simulink model "model"  (R2023b)
settings: Solver=VariableStepAuto  StartTime=0.0  StopTime=10.0  RelTol=1e-3
undefined symbols (not defined in the file): a253, a483c26d3aa4, a58537c8, DiscIntNeverNeededParam, magnitude, Newton, Raphson
libraries: simulink x123, slpidlib x33
(part 2 of 5)

== system model/cfblk92 ==
  cfblk1 : Inport
  cfblk13 : Inport  Port=2
  Action Port : ActionPort  ActionPortLabel=else
  cfblk10 : Sin  TimeSource=Use external signal  SampleTime=0
  cfblk11 : Subsystem
  cfblk12 : Subsystem
  cfblk14 : Delay
  cfblk15 : Delay
  cfblk16 : Delay
  cfblk3 : simulink/Discrete/Transfer Fcn Lead or Lag  PoleZ=0.95  ZeroZ=0.75  ICPrevOutput=0.0  ICPrevInput=0.0  DoSatur=off
  cfblk4 : Product  Inputs=**
  cfblk5 : Sum  Inputs=+-
  cfblk6 : PermuteDimensions
  cfblk7 : Assignment  DiagnosticForDimensions=Warning  IndexOptions=Index vector (dialog)  Indices=1  OutputSizes=1
  cfblk8 : UnaryMinus
  cfblk9 : Product  Inputs=**
  cfblk2 : Outport
  wires:
  cfblk9/1 -> cfblk6/1, cfblk12/4(cfblk10)
  cfblk6/1 -> cfblk5/2, cfblk16/1
  cfblk7/1 -> cfblk11/1(cfblk1)
  cfblk3/1 -> cfblk4/1, cfblk12/3(cfblk9)
  cfblk13/1 -> cfblk8/1
  cfblk12/1(cfblk2) -> cfblk4/2
  cfblk8/1 -> cfblk11/2(cfblk7)
  cfblk5/1 -> cfblk3/1
  cfblk1/1 -> cfblk7/2, cfblk12/2(cfblk8), cfblk9/2
  cfblk11/1(cfblk2) -> cfblk5/1
  cfblk12/2(cfblk11) -> cfblk10/1
  cfblk12/3(cfblk12) -> cfblk2/1
  cfblk4/1 -> cfblk14/1
  cfblk14/1 -> cfblk7/1
  cfblk10/1 -> cfblk15/1
  cfblk15/1 -> cfblk12/1(cfblk1)
  cfblk16/1 -> cfblk9/1

== system model/cfblk93 ==
  cfblk1 : Inport
  cfblk11 : Inport  Port=2
  Action Port : ActionPort  ActionPortLabel=if(u1 >= 0)
  cfblk10 : Subsystem
  cfblk12 : Delay
  cfblk13 : Delay
  cfblk14 : Delay
  cfblk3 : simulink/Discrete/Transfer Fcn Lead or Lag  PoleZ=0.95  ZeroZ=0.75  ICPrevOutput=0.0  ICPrevInput=0.0  DoSatur=off
  cfblk4 : DiscreteZeroPole  Poles=[0 0.5]  Gain=1  SampleTime=-1
  cfblk5 : Product  Inputs=**
  cfblk6 : Sqrt
  cfblk7 : Subsystem
  cfblk8 : Subsystem
  cfblk9 : Subsystem
  cfblk2 : Outport
  wires:
  cfblk3/1 -> cfblk7/1(cfblk1)
  cfblk8/1(cfblk2) -> cfblk6/1
  cfblk5/1 -> cfblk3/1
  cfblk6/1 -> cfblk4/1, cfblk10/3(cfblk12), cfblk14/1
  cfblk7/1(cfblk2) -> cfblk8/1(cfblk1), cfblk10/2(cfblk11)
  cfblk9/1(cfblk2) -> cfblk2/1
  cfblk1/1 -> cfblk5/1, cfblk10/4(cfblk13)
  cfblk11/1 -> cfblk8/2(cfblk13)
  cfblk8/2(cfblk15) -> cfblk10/1(cfblk1), cfblk9/1(cfblk1)
  cfblk10/1(cfblk2) -> cfblk9/2(cfblk12), cfblk13/1
  cfblk4/1 -> cfblk12/1
  cfblk12/1 -> cfblk5/2
  cfblk13/1 -> cfblk8/3(cfblk14)
  cfblk14/1 -> cfblk7/2(cfblk10)

== system model/cfblk94 ==
  cfblk1 : Inport
  cfblk7 : Inport  Port=2
  Action Port : ActionPort  ActionPortLabel=else
  cfblk10 : Delay
  cfblk3 : Delay
  cfblk4 : Sum  Inputs=|++
  cfblk5 : Subsystem
  cfblk6 : Subsystem
  cfblk9 : Delay
  cfblk2 : Outport
  cfblk8 : Outport  Port=2
  wires:
  cfblk1/1 -> cfblk5/1(cfblk1), cfblk6/4(cfblk8)
  cfblk3/1 -> cfblk6/3(cfblk7), cfblk2/1, cfblk9/1, cfblk10/1
  cfblk4/1 -> cfblk3/1
  cfblk6/1(cfblk2) -> cfblk8/1
  cfblk5/1(cfblk2) -> cfblk6/1(cfblk1)
  cfblk5/2(cfblk17) -> cfblk4/1
  cfblk7/1 -> cfblk6/2(cfblk6)
  cfblk9/1 -> cfblk5/2(cfblk16)
  cfblk10/1 -> cfblk4/2

== system model/cfblk95 ==
  cfblk1 : Inport
  cfblk12 : Inport  Port=2
  cfblk13 : Inport  Port=3
  cfblk14 : Inport  Port=4
  Action Port : ActionPort  ActionPortLabel=if(u1 >= 0)
  cfblk10 : Subsystem
  cfblk11 : Subsystem
  cfblk16 : Delay
  cfblk3 : DiscreteZeroPole  Poles=[0 0.5]  Gain=1  SampleTime=-1
  cfblk4 : simulink/Math Operations/MinMax Running Resettable  Function=min  vinit=0.0
  cfblk5 : Sum  Inputs=+
  cfblk6 : DotProduct  OutDataTypeStr=Inherit: Inherit via internal rule
  cfblk7 : Product
  cfblk8 : Constant  Value=[-122431666.096770]  SampleTime=1
  cfblk9 : Constant  Value=[307298168.069237]  SampleTime=1
  cfblk2 : Outport
  cfblk15 : Outport  Port=2
  wires:
  cfblk1/1 -> cfblk7/1
  cfblk10/2(cfblk16) -> cfblk2/1
  cfblk4/1 -> cfblk7/2, cfblk5/1
  cfblk6/1 -> cfblk11/1(cfblk1)
  cfblk8/1 -> cfblk11/2(cfblk8)
  cfblk7/1 -> cfblk6/2
  cfblk11/1(cfblk2) -> cfblk10/1(cfblk1)
  cfblk13/1 -> cfblk10/2(cfblk13)
  cfblk12/1 -> cfblk10/3(cfblk14)
  cfblk3/1 -> cfblk10/4(cfblk15)
  cfblk11/2(cfblk9) -> cfblk15/1
  cfblk5/1 -> cfblk3/1
  cfblk9/1 -> cfblk4/1
  cfblk14/1 -> cfblk4/2
  cfblk10/1(cfblk2) -> cfblk16/1
  cfblk16/1 -> cfblk6/1

== system model/cfblk96 ==
  cfblk1 : Inport
  Action Port : ActionPort  ActionPortLabel=else
  cfblk10 : Subsystem
  cfblk{11..16} (6 alike) : Delay
  cfblk3 : Rounding
  cfblk4 : Subsystem
  cfblk5 : Subsystem
  cfblk6 : Subsystem
  cfblk7 : Subsystem
  cfblk8 : Subsystem
  cfblk9 : Subsystem
  cfblk2 : Outport
  wires:
  cfblk9/1(cfblk2) -> cfblk4/1(cfblk1)
  cfblk6/1(cfblk2) -> cfblk9/1(cfblk1)
  cfblk3/1 -> cfblk7/1(cfblk1)
  cfblk1/1 -> cfblk5/1(cfblk1), cfblk10/3(cfblk8)
  cfblk5/1(cfblk2) -> cfblk10/1(cfblk1), cfblk2/1
  cfblk10/1(cfblk2) -> cfblk6/1(cfblk1)
  cfblk10/2(cfblk10) -> cfblk6/2(cfblk15)
  cfblk9/2(cfblk14) -> cfblk8/2(cfblk6), cfblk15/1
  cfblk6/2(cfblk16) -> cfblk4/2(cfblk14)
  cfblk4/2(cfblk16) -> cfblk8/1(cfblk1), cfblk14/1
  cfblk4/1(cfblk2) -> cfblk11/1
  cfblk11/1 -> cfblk5/2(cfblk12)
  cfblk8/1(cfblk2) -> cfblk12/1
  cfblk12/1 -> cfblk10/2(cfblk7)
  cfblk8/2(cfblk7) -> cfblk13/1
  cfblk13/1 -> cfblk4/3(cfblk15)
  cfblk14/1 -> cfblk10/4(cfblk9)
  cfblk15/1 -> cfblk5/3(cfblk13)
  cfblk7/1(cfblk2) -> cfblk16/1
  cfblk16/1 -> cfblk3/1

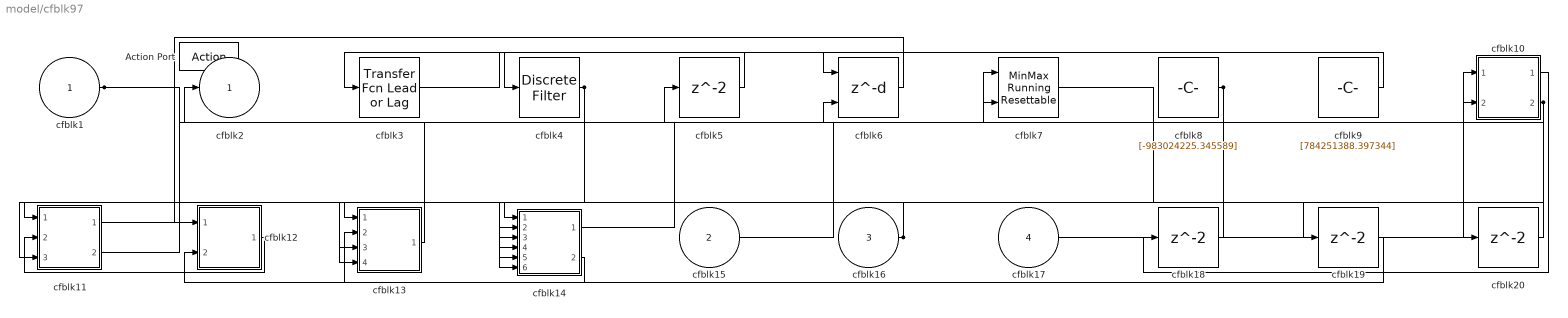
== system model/cfblk97 ==
  cfblk1 : Inport
  cfblk15 : Inport  Port=2
  cfblk16 : Inport  Port=3
  cfblk17 : Inport  Port=4
  Action Port : ActionPort  ActionPortLabel=if(u1 >= 0)
  cfblk10 : Subsystem
  cfblk11 : Subsystem
  cfblk12 : Subsystem
  cfblk13 : Subsystem
  cfblk14 : Subsystem
  cfblk{5,18..20} (4 alike) : Delay
  cfblk3 : simulink/Discrete/Transfer Fcn Lead or Lag  PoleZ=0.95  ZeroZ=0.75  ICPrevOutput=0.0  ICPrevInput=0.0  DoSatur=off
  cfblk4 : DiscreteFilter
  cfblk6 : Delay  DelayLengthSource=Input port
      settings: InputPortMap=u0,p1
  cfblk7 : simulink/Math Operations/MinMax Running Resettable  Function=min  vinit=0.0
  cfblk8 : Constant  Value=[-983024225.345589]  SampleTime=1
  cfblk9 : Constant  Value=[784251388.397344]  SampleTime=1
  cfblk2 : Outport
  wires:
  cfblk14/1(cfblk2) -> cfblk10/1(cfblk1)
  cfblk13/1(cfblk2) -> cfblk2/1
  cfblk6/1 -> cfblk12/1(cfblk1)
  cfblk9/1 -> cfblk4/1
  cfblk17/1 -> cfblk10/2(cfblk9)
  cfblk10/2(cfblk10) -> cfblk5/1, cfblk13/4(cfblk13)
  cfblk3/1 -> cfblk6/1
  cfblk16/1 -> cfblk13/1(cfblk1), cfblk14/3(cfblk13)
  cfblk4/1 -> cfblk11/1(cfblk1), cfblk11/3(cfblk10)
  cfblk8/1 -> cfblk6/2, cfblk14/4(cfblk14), cfblk14/6(cfblk16)
  cfblk5/1 -> cfblk3/1
  cfblk15/1 -> cfblk7/1
  cfblk11/2(cfblk11) -> cfblk7/2
  cfblk14/2(cfblk17) -> cfblk13/2(cfblk11)
  cfblk1/1 -> cfblk13/3(cfblk12), cfblk14/5(cfblk15)
  cfblk12/1(cfblk2) -> cfblk11/2(cfblk9)
  cfblk10/1(cfblk2) -> cfblk18/1
  cfblk18/1 -> cfblk14/1(cfblk1)
  cfblk11/1(cfblk2) -> cfblk19/1
  cfblk19/1 -> cfblk12/2(cfblk8)
  cfblk7/1 -> cfblk20/1
  cfblk20/1 -> cfblk14/2(cfblk12)

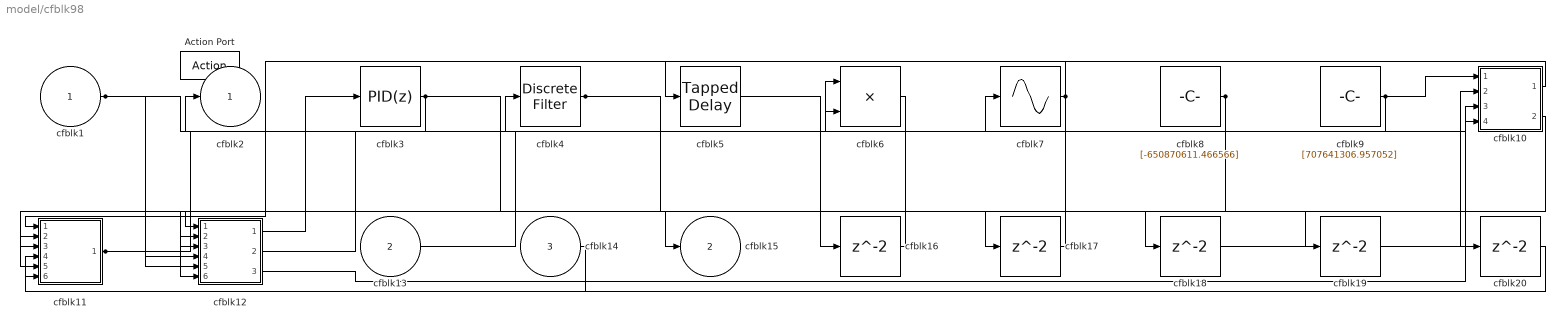
== system model/cfblk98 ==
  cfblk1 : Inport
  cfblk13 : Inport  Port=2
  cfblk14 : Inport  Port=3
  Action Port : ActionPort  ActionPortLabel=else
  cfblk10 : Subsystem
  cfblk11 : Subsystem
  cfblk12 : Subsystem
  cfblk{16..20} (5 alike) : Delay
  cfblk3 : slpidlib/PID Controller  Controller=PID  Form=Parallel  TimeDomain=Discrete-time  UseExternalTs=off  SampleTime=-1  IntegratorMethod=Forward Euler  FilterMethod=Forward Euler  ControllerParametersSource=internal  P=1  I=1  UseKiTs=off  D=0  N=100  UseFilter=on  TunerSelectOption=Transfer Function Based (PID Tuner App)  InitialConditionSource=internal  InitialConditionForIntegrator=0  InitialConditionForFilter=0  DifferentiatorICPrevScaledInput=0  ExternalReset=none  TrackingMode=off  Kt=1  LimitOutput=off  SatLimitsSource=internal  UpperSaturationLimit=inf  LowerSaturationLimit=-inf  LinearizeAsGain=off  AntiWindupMode=none  Kb=1  LimitIntegrator=off  UpperIntegratorSaturationLimit=inf  LowerIntegratorSaturationLimit=-inf  POutMin=[]  POutMax=[]  IOutMin=[]  IOutMax=[]  DOutMin=[]  DOutMax=[]  NOutMin=[]  NOutMax=[]  SumOutMin=[]  SumOutMax=[]  SaturationOutMin=[]  SaturationOutMax=[]  PParamMin=[]  PParamMax=[]  IParamMin=[]  IParamMax=[]  DParamMin=[]  DParamMax=[]  NParamMin=[]  NParamMax=[]  KbParamMin=[]  KbParamMax=[]  KtParamMin=[]  KtParamMax=[]  KbOutMin=[]  KbOutMax=[]  KtOutMin=[]  KtOutMax=[]  IntegratorOutMin=[]  IntegratorOutMax=[]  FilterOutMin=[]  FilterOutMax=[]  SumI1OutMin=[]  SumI1OutMax=[]  SumI2OutMin=[]  SumI2OutMax=[]  SumI3OutMin=[]  SumI3OutMax=[]  SumI4OutMin=[]  SumI4OutMax=[]  SumDOutMin=[]  SumDOutMax=[]  DifferentiatorOutMin=[]  DifferentiatorOutMax=[]  FilterDiffOutCoefMin=[]  FilterDiffOutCoefMax=[]  ReciprocalOutMin=[]  ReciprocalOutMax=[]  SumDenOutMin=[]  SumDenOutMax=[]  SumNumOutMin=[]  SumNumOutMax=[]  DivideOutMin=[]  DivideOutMax=[]  UdiffTsProdOutMin=[]  UdiffTsProdOutMax=[]  NTsProdOutMin=[]  NTsProdOutMax=[]  UintegralTsProdOutMin=[]  UintegralTsProdOutMax=[]  UngainTsProdOutMin=[]  UngainTsProdOutMax=[]  ClampingZeroOutDataTypeStr=Inherit: Inherit via back propagation  ClampingZeroOutMin=[]  ClampingZeroOutMax=[]  FilterDenConstantOutDataTypeStr=Inherit: Inherit via back propagation  FilterDenConstantOutMin=[]  FilterDenConstantOutMax=[]  PCopyOutDataTypeStr=Inherit: Inherit via back propagation  PCopyOutMin=[]  PCopyOutMax=[]  NCopyOutDataTypeStr=Inherit: Inherit via back propagation  NCopyOutMin=[]  NCopyOutMax=[]  IntegratorContinuousStateAttributes=''  IntegratorStateMustResolveToSignalObject=off  IntegratorRTWStateStorageClass=Auto  FilterContinuousStateAttributes=''  FilterStateMustResolveToSignalObject=off  FilterRTWStateStorageClass=Auto  ParallelPVariant=InternalParameters  IdealPVariant=Disabled  IVariant=InternalParameters  DVariant=InternalParameters  IntegratorVariant=Discrete  SatVariant=Disabled  AWVariant=Passthrough  PCopyVariant=Disabled  TRVariant=Disabled  FdbkBlocksVariant=Forward  IdealPFdbkVariant=Disabled  SatFdbkVariant=Disabled  DerivativeFilterVariant=ForwardEulerFilter  NVariant=InternalParameters  NCopyVariant=Disabled  FilterICVariant=InternalICsFilter  IntegratorICVariant=InternalICs  ExternalResetVariant=Disabled  TRSumVariant=Passthrough  SumFdbkVariant=Disabled  SumVariant=Sum_PID  TsampFilterVariant=InternalTs  TsampNgainVariant=Passthrough  TsampIntegralVariant=Disabled_SignalSpec  ExternalSaturationOutDataTypeStr=Inherit: Same as second input
      settings: LibrarySourceBlock=simulink/Discrete/Discrete PID Controller
  cfblk4 : DiscreteFilter
  cfblk5 : simulink/Discrete/Tapped Delay  vinit=0.0  samptime=-1  NumDelays=1  DelayOrder=Oldest  includeCurrent=off
  cfblk6 : Product
  cfblk7 : Sin  TimeSource=Use external signal  SampleTime=0
  cfblk8 : Constant  Value=[-650870611.466566]  SampleTime=1
  cfblk9 : Constant  Value=[707641306.957052]  SampleTime=1
  cfblk2 : Outport
  cfblk15 : Outport  Port=2
  wires:
  cfblk12/1(cfblk2) -> cfblk3/1
  cfblk10/1(cfblk2) -> cfblk11/1(cfblk1)
  cfblk6/1 -> cfblk15/1
  cfblk13/1 -> cfblk6/1
  cfblk11/1(cfblk2) -> cfblk7/1, cfblk12/4(cfblk13)
  cfblk9/1 -> cfblk10/1(cfblk1), cfblk6/2
  cfblk3/1 -> cfblk2/1, cfblk17/1
  cfblk12/2(cfblk16) -> cfblk4/1
  cfblk8/1 -> cfblk11/3(cfblk12), cfblk12/1(cfblk1), cfblk12/3(cfblk12)
  cfblk7/1 -> cfblk5/1, cfblk12/6(cfblk15)
  cfblk14/1 -> cfblk11/4(cfblk13)
  cfblk4/1 -> cfblk18/1, cfblk19/1
  cfblk10/2(cfblk8) -> cfblk11/5(cfblk14)
  cfblk1/1 -> cfblk10/3(cfblk6), cfblk12/5(cfblk14)
  cfblk5/1 -> cfblk16/1
  cfblk16/1 -> cfblk11/2(cfblk11)
  cfblk17/1 -> cfblk12/2(cfblk11)
  cfblk18/1 -> cfblk10/2(cfblk5)
  cfblk19/1 -> cfblk10/4(cfblk7)
  cfblk12/3(cfblk17) -> cfblk20/1
  cfblk20/1 -> cfblk11/6(cfblk15)

== system model/cfblk99 ==
  cfblk1 : Inport
  Action Port : ActionPort  ActionPortLabel=if(u1 >= 0)
  cfblk{9..14} (6 alike) : Delay
  cfblk3 : DiscreteZeroPole  Poles=[0 0.5]  Gain=1  SampleTime=-1
  cfblk4 : Product  Inputs=*
  cfblk5 : Subsystem
  cfblk6 : Subsystem
  cfblk7 : Subsystem
  cfblk8 : Subsystem
  cfblk2 : Outport
  wires:
  cfblk4/1 -> cfblk6/4(cfblk13), cfblk6/6(cfblk15), cfblk9/1, cfblk10/1
  cfblk5/1(cfblk2) -> cfblk2/1, cfblk8/2(cfblk14), cfblk6/2(cfblk11)
  cfblk7/1(cfblk2) -> cfblk4/1, cfblk6/1(cfblk1)
  cfblk8/1(cfblk2) -> cfblk7/2(cfblk16)
  cfblk6/1(cfblk2) -> cfblk11/1, cfblk12/1
  cfblk8/2(cfblk15) -> cfblk3/1
  cfblk1/1 -> cfblk5/1(cfblk1)
  cfblk3/1 -> cfblk6/5(cfblk14), cfblk13/1
  cfblk8/3(cfblk16) -> cfblk6/3(cfblk12), cfblk14/1
  cfblk9/1 -> cfblk7/1(cfblk1)
  cfblk10/1 -> cfblk8/1(cfblk1)
  cfblk11/1 -> cfblk7/3(cfblk17)
  cfblk12/1 -> cfblk5/4(cfblk12)
  cfblk13/1 -> cfblk5/2(cfblk10)
  cfblk14/1 -> cfblk5/3(cfblk11)

== system model/cfblk100/cfblk10 ==
  cfblk1 : Inport
  cfblk16 : Inport  Port=2
  cfblk10 : simulink/Math Operations/MinMax Running Resettable  Function=min  vinit=0.0
  cfblk11 : Math  Operator=transpose
  cfblk12 : Constant  Value=[636761665.784552]  SampleTime=1
  cfblk13 : Constant  Value=[-211906745.955713]  SampleTime=1
  cfblk14 : Constant  Value=[150860289.272291]  SampleTime=1
  cfblk15 : Constant  Value=[368874745.790174]  SampleTime=1
  cfblk3 : Delay
  cfblk4 : Delay  ShowEnablePort=on
      settings: InputPortMap=u0,e6
  cfblk5 : simulink/Discrete/Difference  ICPrevInput=0.0  OutMin=[]  OutMax=[]  OutDataTypeStr=Inherit: Inherit via back propagation  OutDataType=fixdt(1, 16)  OutScaling=2^-10  DoSatur=off
  cfblk6 : slpidlib/PID Controller  Controller=PID  Form=Parallel  TimeDomain=Discrete-time  UseExternalTs=off  SampleTime=-1  IntegratorMethod=Forward Euler  FilterMethod=Forward Euler  ControllerParametersSource=internal  P=1  I=1  UseKiTs=off  D=0  N=100  UseFilter=on  TunerSelectOption=Transfer Function Based (PID Tuner App)  InitialConditionSource=internal  InitialConditionForIntegrator=0  InitialConditionForFilter=0  DifferentiatorICPrevScaledInput=0  ExternalReset=none  TrackingMode=off  Kt=1  LimitOutput=off  SatLimitsSource=internal  UpperSaturationLimit=inf  LowerSaturationLimit=-inf  LinearizeAsGain=off  AntiWindupMode=none  Kb=1  LimitIntegrator=off  UpperIntegratorSaturationLimit=inf  LowerIntegratorSaturationLimit=-inf  POutMin=[]  POutMax=[]  IOutMin=[]  IOutMax=[]  DOutMin=[]  DOutMax=[]  NOutMin=[]  NOutMax=[]  SumOutMin=[]  SumOutMax=[]  SaturationOutMin=[]  SaturationOutMax=[]  PParamMin=[]  PParamMax=[]  IParamMin=[]  IParamMax=[]  DParamMin=[]  DParamMax=[]  NParamMin=[]  NParamMax=[]  KbParamMin=[]  KbParamMax=[]  KtParamMin=[]  KtParamMax=[]  KbOutMin=[]  KbOutMax=[]  KtOutMin=[]  KtOutMax=[]  IntegratorOutMin=[]  IntegratorOutMax=[]  FilterOutMin=[]  FilterOutMax=[]  SumI1OutMin=[]  SumI1OutMax=[]  SumI2OutMin=[]  SumI2OutMax=[]  SumI3OutMin=[]  SumI3OutMax=[]  SumI4OutMin=[]  SumI4OutMax=[]  SumDOutMin=[]  SumDOutMax=[]  DifferentiatorOutMin=[]  DifferentiatorOutMax=[]  FilterDiffOutCoefMin=[]  FilterDiffOutCoefMax=[]  ReciprocalOutMin=[]  ReciprocalOutMax=[]  SumDenOutMin=[]  SumDenOutMax=[]  SumNumOutMin=[]  SumNumOutMax=[]  DivideOutMin=[]  DivideOutMax=[]  UdiffTsProdOutMin=[]  UdiffTsProdOutMax=[]  NTsProdOutMin=[]  NTsProdOutMax=[]  UintegralTsProdOutMin=[]  UintegralTsProdOutMax=[]  UngainTsProdOutMin=[]  UngainTsProdOutMax=[]  ClampingZeroOutDataTypeStr=Inherit: Inherit via back propagation  ClampingZeroOutMin=[]  ClampingZeroOutMax=[]  FilterDenConstantOutDataTypeStr=Inherit: Inherit via back propagation  FilterDenConstantOutMin=[]  FilterDenConstantOutMax=[]  PCopyOutDataTypeStr=Inherit: Inherit via back propagation  PCopyOutMin=[]  PCopyOutMax=[]  NCopyOutDataTypeStr=Inherit: Inherit via back propagation  NCopyOutMin=[]  NCopyOutMax=[]  IntegratorContinuousStateAttributes=''  IntegratorStateMustResolveToSignalObject=off  IntegratorRTWStateStorageClass=Auto  FilterContinuousStateAttributes=''  FilterStateMustResolveToSignalObject=off  FilterRTWStateStorageClass=Auto  ParallelPVariant=InternalParameters  IdealPVariant=Disabled  IVariant=InternalParameters  DVariant=InternalParameters  IntegratorVariant=Discrete  SatVariant=Disabled  AWVariant=Passthrough  PCopyVariant=Disabled  TRVariant=Disabled  FdbkBlocksVariant=Forward  IdealPFdbkVariant=Disabled  SatFdbkVariant=Disabled  DerivativeFilterVariant=ForwardEulerFilter  NVariant=InternalParameters  NCopyVariant=Disabled  FilterICVariant=InternalICsFilter  IntegratorICVariant=InternalICs  ExternalResetVariant=Disabled  TRSumVariant=Passthrough  SumFdbkVariant=Disabled  SumVariant=Sum_PID  TsampFilterVariant=InternalTs  TsampNgainVariant=Passthrough  TsampIntegralVariant=Disabled_SignalSpec  ExternalSaturationOutDataTypeStr=Inherit: Same as second input
      settings: LibrarySourceBlock=simulink/Discrete/Discrete PID Controller
  cfblk7 : simulink/Discrete/Tapped Delay  vinit=0.0  samptime=-1  NumDelays=1  DelayOrder=Oldest  includeCurrent=off
  cfblk8 : ComplexToRealImag
  cfblk9 : simulink/Math Operations/Slider Gain  gain=1  low=0  high=2
  cfblk2 : Outport
  cfblk17 : Outport  Port=2
  wires:
  cfblk4/1 -> cfblk8/1
  cfblk7/1 -> cfblk6/1
  cfblk15/1 -> cfblk7/1
  cfblk1/1 -> cfblk9/1
  cfblk16/1 -> cfblk4/1
  cfblk8/1 -> cfblk17/1
  cfblk11/1 -> cfblk2/1
  cfblk12/1 -> cfblk4/2
  cfblk6/1 -> cfblk5/1
  cfblk8/2 -> cfblk10/1
  cfblk9/1 -> cfblk3/1
  cfblk3/1 -> cfblk11/1
  cfblk14/1 -> cfblk10/2

== system model/cfblk100/cfblk11 ==
  cfblk1 : Inport
  cfblk10 : Inport  Port=2
  cfblk11 : Inport  Port=3
  cfblk12 : Inport  Port=4
  cfblk13 : Inport  Port=5
  cfblk14 : Inport  Port=6
  cfblk3 : Product  Inputs=**
  cfblk4 : Sum  Inputs=+-
  cfblk5 : Polyval  Coefs=[ +2.081618890e-019, -1.441693666e-014, +4.719686976e-010, -8.536869453e-006, +1.621573104e-001, -8.087801117e+001 ]
  cfblk6 : Assignment  DiagnosticForDimensions=Warning  IndexOptions=Index vector (dialog)  Indices=1  OutputSizes=1
  cfblk7 : PermuteDimensions
  cfblk8 : Constant  Value=[971807182.995786]  SampleTime=1
  cfblk9 : Constant  Value=[534137876.527184]  SampleTime=1
  cfblk2 : Outport
  cfblk15 : Outport  Port=2
  wires:
  cfblk1/1 -> cfblk7/1
  cfblk6/1 -> cfblk3/1
  cfblk8/1 -> cfblk15/1
  cfblk10/1 -> cfblk3/2
  cfblk5/1 -> cfblk2/1
  cfblk7/1 -> cfblk6/1
  cfblk11/1 -> cfblk4/1
  cfblk3/1 -> cfblk4/2
  cfblk4/1 -> cfblk5/1
  cfblk14/1 -> cfblk6/2

== system model/cfblk100/cfblk12 ==
  cfblk1 : Inport
  cfblk6 : Inport  Port=2
  cfblk7 : Inport  Port=3
  cfblk8 : Inport  Port=4
  cfblk3 : MinMax
  cfblk4 : Constant  Value=[120528931.292564]  SampleTime=1
  cfblk5 : Constant  Value=[473078262.944689]  SampleTime=1
  cfblk2 : Outport
  wires:
  cfblk3/1 -> cfblk2/1
  cfblk6/1 -> cfblk3/1

== system model/cfblk100/cfblk13 ==
  cfblk1 : Inport
  cfblk14 : Inport  Port=2
  cfblk15 : Inport  Port=3
  cfblk16 : Inport  Port=4
  cfblk17 : Inport  Port=5
  cfblk10 : Constant  Value=[-106226316.947558]  SampleTime=1
  cfblk11 : Constant  Value=[-816921342.665887]  SampleTime=1
  cfblk12 : Constant  Value=[662496764.095145]  SampleTime=1
  cfblk13 : Constant  Value=[-996755298.723096]  SampleTime=1
  cfblk3 : Bias  Bias=[632524479.688455]  SaturateOnIntegerOverflow=off
  cfblk4 : Abs  SaturateOnIntegerOverflow=off
  cfblk5 : PermuteDimensions
  cfblk6 : Abs  SaturateOnIntegerOverflow=off
  cfblk7 : Sum  Inputs=+-
  cfblk8 : Rounding
  cfblk9 : Product  Inputs=*
  cfblk2 : Outport
  wires:
  cfblk15/1 -> cfblk3/1
  cfblk12/1 -> cfblk4/1
  cfblk5/1 -> cfblk2/1
  cfblk17/1 -> cfblk5/1
  cfblk16/1 -> cfblk6/1
  cfblk11/1 -> cfblk9/1
  cfblk13/1 -> cfblk7/1
  cfblk10/1 -> cfblk8/1
  cfblk4/1 -> cfblk7/2

== system model/cfblk65/cfblk13 ==
  cfblk1 : Inport
  cfblk12 : Inport  Port=2
  cfblk13 : Inport  Port=3
  cfblk10 : Gain  Gain=[31942379.189756]
  cfblk11 : MinMax  Inputs=2
  cfblk16 : Delay  SampleTime=1
  cfblk3 : Delay  DelayLengthSource=Input port  SampleTime=1
      settings: InputPortMap=u0,p1
  cfblk4 : PropagationDelay  SampleTime=1
  cfblk5 : DiscreteStateSpace
  cfblk6 : UnitDelay  HasFrameUpgradeWarning=on
  cfblk7 : slpidlib/PID Controller  Controller=PID  Form=Parallel  TimeDomain=Discrete-time  UseExternalTs=off  SampleTime=1  IntegratorMethod=Forward Euler  FilterMethod=Forward Euler  ControllerParametersSource=internal  P=1  I=1  UseKiTs=off  D=0  N=100  UseFilter=on  TunerSelectOption=Transfer Function Based (PID Tuner App)  InitialConditionSource=internal  InitialConditionForIntegrator=0  InitialConditionForFilter=0  DifferentiatorICPrevScaledInput=0  ExternalReset=none  TrackingMode=off  Kt=1  LimitOutput=off  SatLimitsSource=internal  UpperSaturationLimit=inf  LowerSaturationLimit=-inf  LinearizeAsGain=off  AntiWindupMode=none  Kb=1  LimitIntegrator=off  UpperIntegratorSaturationLimit=inf  LowerIntegratorSaturationLimit=-inf  POutMin=[]  POutMax=[]  IOutMin=[]  IOutMax=[]  DOutMin=[]  DOutMax=[]  NOutMin=[]  NOutMax=[]  SumOutMin=[]  SumOutMax=[]  SaturationOutMin=[]  SaturationOutMax=[]  PParamMin=[]  PParamMax=[]  IParamMin=[]  IParamMax=[]  DParamMin=[]  DParamMax=[]  NParamMin=[]  NParamMax=[]  KbParamMin=[]  KbParamMax=[]  KtParamMin=[]  KtParamMax=[]  KbOutMin=[]  KbOutMax=[]  KtOutMin=[]  KtOutMax=[]  IntegratorOutMin=[]  IntegratorOutMax=[]  FilterOutMin=[]  FilterOutMax=[]  SumI1OutMin=[]  SumI1OutMax=[]  SumI2OutMin=[]  SumI2OutMax=[]  SumI3OutMin=[]  SumI3OutMax=[]  SumI4OutMin=[]  SumI4OutMax=[]  SumDOutMin=[]  SumDOutMax=[]  DifferentiatorOutMin=[]  DifferentiatorOutMax=[]  FilterDiffOutCoefMin=[]  FilterDiffOutCoefMax=[]  ReciprocalOutMin=[]  ReciprocalOutMax=[]  SumDenOutMin=[]  SumDenOutMax=[]  SumNumOutMin=[]  SumNumOutMax=[]  DivideOutMin=[]  DivideOutMax=[]  UdiffTsProdOutMin=[]  UdiffTsProdOutMax=[]  NTsProdOutMin=[]  NTsProdOutMax=[]  UintegralTsProdOutMin=[]  UintegralTsProdOutMax=[]  UngainTsProdOutMin=[]  UngainTsProdOutMax=[]  ClampingZeroOutDataTypeStr=Inherit: Inherit via back propagation  ClampingZeroOutMin=[]  ClampingZeroOutMax=[]  FilterDenConstantOutDataTypeStr=Inherit: Inherit via back propagation  FilterDenConstantOutMin=[]  FilterDenConstantOutMax=[]  PCopyOutDataTypeStr=Inherit: Inherit via back propagation  PCopyOutMin=[]  PCopyOutMax=[]  NCopyOutDataTypeStr=Inherit: Inherit via back propagation  NCopyOutMin=[]  NCopyOutMax=[]  IntegratorContinuousStateAttributes=''  IntegratorStateMustResolveToSignalObject=off  IntegratorRTWStateStorageClass=Auto  FilterContinuousStateAttributes=''  FilterStateMustResolveToSignalObject=off  FilterRTWStateStorageClass=Auto  ParallelPVariant=InternalParameters  IdealPVariant=Disabled  IVariant=InternalParameters  DVariant=InternalParameters  IntegratorVariant=Discrete  SatVariant=Disabled  AWVariant=Passthrough  PCopyVariant=Disabled  TRVariant=Disabled  FdbkBlocksVariant=Forward  IdealPFdbkVariant=Disabled  SatFdbkVariant=Disabled  DerivativeFilterVariant=ForwardEulerFilter  NVariant=InternalParameters  NCopyVariant=Disabled  FilterICVariant=InternalICsFilter  IntegratorICVariant=InternalICs  ExternalResetVariant=Disabled  TRSumVariant=Passthrough  SumFdbkVariant=Disabled  SumVariant=Sum_PID  TsampFilterVariant=InternalTs  TsampNgainVariant=Passthrough  TsampIntegralVariant=Disabled_SignalSpec  ExternalSaturationOutDataTypeStr=Inherit: Same as second input
      settings: LibrarySourceBlock=simulink/Discrete/Discrete PID Controller
  cfblk8 : Sum  Inputs=|++
  cfblk9 : Sqrt
  cfblk2 : Outport
  cfblk14 : Outport  Port=2
  cfblk15 : Outport  Port=3
  wires:
  cfblk7/1 -> cfblk2/1, cfblk4/2
  cfblk12/1 -> cfblk10/1
  cfblk5/1 -> cfblk7/1, cfblk3/2
  cfblk8/1 -> cfblk11/1
  cfblk4/1 -> cfblk15/1
  cfblk9/1 -> cfblk11/2
  cfblk6/1 -> cfblk14/1
  cfblk1/1 -> cfblk5/1
  cfblk13/1 -> cfblk3/1
  cfblk3/1 -> cfblk8/2, cfblk9/1, cfblk4/1
  cfblk10/1 -> cfblk6/1
  cfblk11/1 -> cfblk16/1
  cfblk16/1 -> cfblk8/1

== system model/cfblk65/cfblk14 ==
  cfblk1 : Inport
  cfblk10 : Inport  Port=2
  cfblk11 : Inport  Port=3
  cfblk12 : Inport  Port=4
  cfblk3 : slpidlib/PID Controller  Controller=PID  Form=Parallel  TimeDomain=Discrete-time  UseExternalTs=off  SampleTime=1  IntegratorMethod=Forward Euler  FilterMethod=Forward Euler  ControllerParametersSource=internal  P=1  I=1  UseKiTs=off  D=0  N=100  UseFilter=on  TunerSelectOption=Transfer Function Based (PID Tuner App)  InitialConditionSource=internal  InitialConditionForIntegrator=0  InitialConditionForFilter=0  DifferentiatorICPrevScaledInput=0  ExternalReset=none  TrackingMode=off  Kt=1  LimitOutput=off  SatLimitsSource=internal  UpperSaturationLimit=inf  LowerSaturationLimit=-inf  LinearizeAsGain=off  AntiWindupMode=none  Kb=1  LimitIntegrator=off  UpperIntegratorSaturationLimit=inf  LowerIntegratorSaturationLimit=-inf  POutMin=[]  POutMax=[]  IOutMin=[]  IOutMax=[]  DOutMin=[]  DOutMax=[]  NOutMin=[]  NOutMax=[]  SumOutMin=[]  SumOutMax=[]  SaturationOutMin=[]  SaturationOutMax=[]  PParamMin=[]  PParamMax=[]  IParamMin=[]  IParamMax=[]  DParamMin=[]  DParamMax=[]  NParamMin=[]  NParamMax=[]  KbParamMin=[]  KbParamMax=[]  KtParamMin=[]  KtParamMax=[]  KbOutMin=[]  KbOutMax=[]  KtOutMin=[]  KtOutMax=[]  IntegratorOutMin=[]  IntegratorOutMax=[]  FilterOutMin=[]  FilterOutMax=[]  SumI1OutMin=[]  SumI1OutMax=[]  SumI2OutMin=[]  SumI2OutMax=[]  SumI3OutMin=[]  SumI3OutMax=[]  SumI4OutMin=[]  SumI4OutMax=[]  SumDOutMin=[]  SumDOutMax=[]  DifferentiatorOutMin=[]  DifferentiatorOutMax=[]  FilterDiffOutCoefMin=[]  FilterDiffOutCoefMax=[]  ReciprocalOutMin=[]  ReciprocalOutMax=[]  SumDenOutMin=[]  SumDenOutMax=[]  SumNumOutMin=[]  SumNumOutMax=[]  DivideOutMin=[]  DivideOutMax=[]  UdiffTsProdOutMin=[]  UdiffTsProdOutMax=[]  NTsProdOutMin=[]  NTsProdOutMax=[]  UintegralTsProdOutMin=[]  UintegralTsProdOutMax=[]  UngainTsProdOutMin=[]  UngainTsProdOutMax=[]  ClampingZeroOutDataTypeStr=Inherit: Inherit via back propagation  ClampingZeroOutMin=[]  ClampingZeroOutMax=[]  FilterDenConstantOutDataTypeStr=Inherit: Inherit via back propagation  FilterDenConstantOutMin=[]  FilterDenConstantOutMax=[]  PCopyOutDataTypeStr=Inherit: Inherit via back propagation  PCopyOutMin=[]  PCopyOutMax=[]  NCopyOutDataTypeStr=Inherit: Inherit via back propagation  NCopyOutMin=[]  NCopyOutMax=[]  IntegratorContinuousStateAttributes=''  IntegratorStateMustResolveToSignalObject=off  IntegratorRTWStateStorageClass=Auto  FilterContinuousStateAttributes=''  FilterStateMustResolveToSignalObject=off  FilterRTWStateStorageClass=Auto  ParallelPVariant=InternalParameters  IdealPVariant=Disabled  IVariant=InternalParameters  DVariant=InternalParameters  IntegratorVariant=Discrete  SatVariant=Disabled  AWVariant=Passthrough  PCopyVariant=Disabled  TRVariant=Disabled  FdbkBlocksVariant=Forward  IdealPFdbkVariant=Disabled  SatFdbkVariant=Disabled  DerivativeFilterVariant=ForwardEulerFilter  NVariant=InternalParameters  NCopyVariant=Disabled  FilterICVariant=InternalICsFilter  IntegratorICVariant=InternalICs  ExternalResetVariant=Disabled  TRSumVariant=Passthrough  SumFdbkVariant=Disabled  SumVariant=Sum_PID  TsampFilterVariant=InternalTs  TsampNgainVariant=Passthrough  TsampIntegralVariant=Disabled_SignalSpec  ExternalSaturationOutDataTypeStr=Inherit: Same as second input
      settings: LibrarySourceBlock=simulink/Discrete/Discrete PID Controller
  cfblk4 : simulink/Discrete/Transfer Fcn First Order  PoleZ=0.95  ICPrevOutput=0.0  DoSatur=off
  cfblk5 : DiscreteTransferFcn  SampleTime=1
  cfblk6 : Delay  ShowEnablePort=on  SampleTime=1
      settings: InputPortMap=u0,e6
  cfblk7 : simulink/Discrete/Transfer Fcn First Order  PoleZ=0.95  ICPrevOutput=0.0  DoSatur=off
  cfblk8 : Gain  Gain=[-907888824.165032]
  cfblk9 : Constant  Value=[263984584.005114]  SampleTime=1
  cfblk2 : Outport
  cfblk13 : Outport  Port=2
  cfblk14 : Outport  Port=3
  cfblk15 : Outport  Port=4
  wires:
  cfblk3/1 -> cfblk2/1
  cfblk7/1 -> cfblk8/1
  cfblk11/1 -> cfblk6/1
  cfblk9/1 -> cfblk5/1
  cfblk8/1 -> cfblk6/2
  cfblk6/1 -> cfblk13/1
  cfblk1/1 -> cfblk15/1
  cfblk12/1 -> cfblk14/1
  cfblk5/1 -> cfblk4/1
  cfblk10/1 -> cfblk7/1
  cfblk4/1 -> cfblk3/1

== system model/cfblk66/cfblk10 ==
  cfblk1 : Inport
  cfblk3 : Delay  SampleTime=1
  cfblk4 : Sqrt
  cfblk5 : Math  Operator=conj
  cfblk6 : simulink/Math Operations/MinMax Running Resettable  Function=min  vinit=0.0
  cfblk8 : Delay  SampleTime=1
  cfblk2 : Outport
  cfblk7 : Outport  Port=2
  wires:
  cfblk4/1 -> cfblk7/1
  cfblk1/1 -> cfblk2/1, cfblk6/2
  cfblk6/1 -> cfblk5/1
  cfblk5/1 -> cfblk3/1, cfblk4/1
  cfblk3/1 -> cfblk8/1
  cfblk8/1 -> cfblk6/1

== system model/cfblk66/cfblk11 ==
  cfblk1 : Inport
  cfblk10 : Sqrt
  cfblk11 : Product
  cfblk12 : Sum  Inputs=|++
  cfblk13 : Rounding
  cfblk17 : Delay  SampleTime=1
  cfblk3 : PropagationDelay  SampleTime=1
  cfblk4 : DiscreteFilter  SampleTime=1
  cfblk5 : simulink/Discrete/Transfer Fcn Real Zero  ZeroZ=0.75  ICPrevInput=0.0  DoSatur=off
  cfblk6 : simulink/Discrete/Transfer Fcn First Order  PoleZ=0.95  ICPrevOutput=0.0  DoSatur=off
  cfblk7 : Sqrt
  cfblk8 : Reshape
  cfblk9 : Product  Inputs=*
  cfblk2 : Outport
  cfblk14 : Outport  Port=2
  cfblk15 : Outport  Port=3
  cfblk16 : Outport  Port=4
  wires:
  cfblk5/1 -> cfblk3/1
  cfblk10/1 -> cfblk16/1
  cfblk7/1 -> cfblk6/1
  cfblk8/1 -> cfblk10/1, cfblk15/1, cfblk17/1
  cfblk3/1 -> cfblk2/1, cfblk8/1
  cfblk6/1 -> cfblk9/1, cfblk14/1, cfblk5/1
  cfblk13/1 -> cfblk7/1
  cfblk9/1 -> cfblk4/1, cfblk12/2
  cfblk4/1 -> cfblk12/1
  cfblk12/1 -> cfblk11/1
  cfblk11/1 -> cfblk3/2
  cfblk1/1 -> cfblk13/1
  cfblk17/1 -> cfblk11/2

== system model/cfblk66/cfblk9 ==
  cfblk1 : Inport
  cfblk12 : Inport  Port=2
  cfblk13 : Inport  Port=3
  cfblk14 : Inport  Port=4
  cfblk15 : Inport  Port=5
  cfblk10 : Constant  Value=[-598054874.618713]  SampleTime=1
  cfblk11 : Constant  Value=[-182307291.985765]  SampleTime=1
  cfblk17 : Delay  SampleTime=1
  cfblk3 : Delay  DelayLengthSource=Input port  SampleTime=1
      settings: InputPortMap=u0,p1
  cfblk4 : DiscreteStateSpace
  cfblk5 : Sqrt
  cfblk6 : Math  Operator=magnitude^2
  cfblk7 : Product  Inputs=**
  cfblk8 : Sum  Inputs=-+
  cfblk9 : Constant  Value=[-430698735.578265]  SampleTime=1
  cfblk2 : Outport
  cfblk16 : Outport  Port=2
  wires:
  cfblk15/1 -> cfblk16/1
  cfblk9/1 -> cfblk4/1
  cfblk1/1 -> cfblk2/1
  cfblk13/1 -> cfblk3/1
  cfblk8/1 -> cfblk7/1
  cfblk3/1 -> cfblk6/1
  cfblk6/1 -> cfblk8/1
  cfblk5/1 -> cfblk7/2
  cfblk12/1 -> cfblk5/1
  cfblk11/1 -> cfblk8/2
  cfblk7/1 -> cfblk17/1
  cfblk17/1 -> cfblk3/2

== system model/cfblk67/cfblk10 ==
  cfblk1 : Inport
  cfblk9 : Inport  Port=2
  cfblk10 : Inport  Port=3
  cfblk11 : Inport  Port=4
  cfblk12 : Inport  Port=5
  cfblk15 : Delay  SampleTime=1
  cfblk3 : DiscreteFilter  SampleTime=1
  cfblk4 : Sqrt
  cfblk5 : Sum  Inputs=+-
  cfblk6 : Product  Inputs=*
  cfblk7 : Polyval  Coefs=[ +2.081618890e-019, -1.441693666e-014, +4.719686976e-010, -8.536869453e-006, +1.621573104e-001, -8.087801117e+001 ]
  cfblk8 : Constant  Value=[-479611448.539397]  SampleTime=1
  cfblk2 : Outport
  cfblk13 : Outport  Port=2
  cfblk14 : Outport  Port=3
  wires:
  cfblk11/1 -> cfblk6/1
  cfblk6/1 -> cfblk2/1
  cfblk10/1 -> cfblk4/1
  cfblk12/1 -> cfblk13/1
  cfblk8/1 -> cfblk14/1
  cfblk9/1 -> cfblk5/1
  cfblk3/1 -> cfblk5/2
  cfblk5/1 -> cfblk7/1
  cfblk7/1 -> cfblk15/1
  cfblk15/1 -> cfblk3/1

== system model/cfblk67/cfblk11 ==
  cfblk1 : Inport
  cfblk7 : Inport  Port=2
  cfblk3 : DiscreteFir  SampleTime=1
  cfblk4 : Sum  Inputs=+
  cfblk5 : Trigonometry
  cfblk6 : Constant  Value=[49582587.309329]  SampleTime=1
  cfblk8 : Delay  SampleTime=1
  cfblk2 : Outport
  wires:
  cfblk4/1 -> cfblk2/1
  cfblk3/1 -> cfblk5/1
  cfblk1/1 -> cfblk4/1
  cfblk5/1 -> cfblk8/1
  cfblk8/1 -> cfblk3/1

== system model/cfblk68/cfblk12 ==
  cfblk1 : Inport
  cfblk10 : Inport  Port=2
  cfblk11 : Inport  Port=3
  cfblk12 : Inport  Port=4
  cfblk3 : simulink/Discrete/Transfer Fcn Lead or Lag  PoleZ=0.95  ZeroZ=0.75  ICPrevOutput=0.0  ICPrevInput=0.0  DoSatur=off
  cfblk4 : UnitDelay  HasFrameUpgradeWarning=on
  cfblk5 : Polyval  Coefs=[ +2.081618890e-019, -1.441693666e-014, +4.719686976e-010, -8.536869453e-006, +1.621573104e-001, -8.087801117e+001 ]
  cfblk6 : Polyval  Coefs=[ +2.081618890e-019, -1.441693666e-014, +4.719686976e-010, -8.536869453e-006, +1.621573104e-001, -8.087801117e+001 ]
  cfblk7 : Sum  Inputs=+
  cfblk8 : Constant  Value=[-879986801.323946]  SampleTime=1
  cfblk9 : Constant  Value=[-235399529.876834]  SampleTime=1
  cfblk2 : Outport
  cfblk13 : Outport  Port=2
  wires:
  cfblk4/1 -> cfblk6/1
  cfblk11/1 -> cfblk5/1
  cfblk6/1 -> cfblk13/1
  cfblk1/1 -> cfblk3/1
  cfblk9/1 -> cfblk4/1
  cfblk12/1 -> cfblk2/1
  cfblk3/1 -> cfblk7/1

== system model/cfblk68/cfblk13 ==
  cfblk1 : Inport
  cfblk7 : Inport  Port=2
  cfblk8 : Inport  Port=3
  cfblk10 : Delay  SampleTime=1
  cfblk3 : DiscreteZeroPole  Poles=[0 0.5]  Gain=1
  cfblk4 : Delay  ShowEnablePort=on  SampleTime=1
      settings: InputPortMap=u0,e6
  cfblk5 : simulink/Math Operations/MinMax Running Resettable  Function=min  vinit=0.0
  cfblk6 : Constant  Value=[-700906495.696172]  SampleTime=1
  cfblk2 : Outport
  cfblk9 : Outport  Port=2
  wires:
  cfblk7/1 -> cfblk5/1
  cfblk3/1 -> cfblk9/1
  cfblk6/1 -> cfblk3/1
  cfblk8/1 -> cfblk2/1
  cfblk1/1 -> cfblk4/2
  cfblk4/1 -> cfblk5/2
  cfblk5/1 -> cfblk10/1
  cfblk10/1 -> cfblk4/1

== system model/cfblk69/cfblk7 ==
  cfblk1 : Inport
  cfblk9 : Inport  Port=2
  cfblk10 : Inport  Port=3
  cfblk12 : Delay  SampleTime=1
  cfblk3 : simulink/Discrete/Transfer Fcn Lead or Lag  PoleZ=0.95  ZeroZ=0.75  ICPrevOutput=0.0  ICPrevInput=0.0  DoSatur=off
  cfblk4 : slpidlib/PID Controller  Controller=PID  Form=Parallel  TimeDomain=Discrete-time  UseExternalTs=off  SampleTime=1  IntegratorMethod=Forward Euler  FilterMethod=Forward Euler  ControllerParametersSource=internal  P=1  I=1  UseKiTs=off  D=0  N=100  UseFilter=on  TunerSelectOption=Transfer Function Based (PID Tuner App)  InitialConditionSource=internal  InitialConditionForIntegrator=0  InitialConditionForFilter=0  DifferentiatorICPrevScaledInput=0  ExternalReset=none  TrackingMode=off  Kt=1  LimitOutput=off  SatLimitsSource=internal  UpperSaturationLimit=inf  LowerSaturationLimit=-inf  LinearizeAsGain=off  AntiWindupMode=none  Kb=1  LimitIntegrator=off  UpperIntegratorSaturationLimit=inf  LowerIntegratorSaturationLimit=-inf  POutMin=[]  POutMax=[]  IOutMin=[]  IOutMax=[]  DOutMin=[]  DOutMax=[]  NOutMin=[]  NOutMax=[]  SumOutMin=[]  SumOutMax=[]  SaturationOutMin=[]  SaturationOutMax=[]  PParamMin=[]  PParamMax=[]  IParamMin=[]  IParamMax=[]  DParamMin=[]  DParamMax=[]  NParamMin=[]  NParamMax=[]  KbParamMin=[]  KbParamMax=[]  KtParamMin=[]  KtParamMax=[]  KbOutMin=[]  KbOutMax=[]  KtOutMin=[]  KtOutMax=[]  IntegratorOutMin=[]  IntegratorOutMax=[]  FilterOutMin=[]  FilterOutMax=[]  SumI1OutMin=[]  SumI1OutMax=[]  SumI2OutMin=[]  SumI2OutMax=[]  SumI3OutMin=[]  SumI3OutMax=[]  SumI4OutMin=[]  SumI4OutMax=[]  SumDOutMin=[]  SumDOutMax=[]  DifferentiatorOutMin=[]  DifferentiatorOutMax=[]  FilterDiffOutCoefMin=[]  FilterDiffOutCoefMax=[]  ReciprocalOutMin=[]  ReciprocalOutMax=[]  SumDenOutMin=[]  SumDenOutMax=[]  SumNumOutMin=[]  SumNumOutMax=[]  DivideOutMin=[]  DivideOutMax=[]  UdiffTsProdOutMin=[]  UdiffTsProdOutMax=[]  NTsProdOutMin=[]  NTsProdOutMax=[]  UintegralTsProdOutMin=[]  UintegralTsProdOutMax=[]  UngainTsProdOutMin=[]  UngainTsProdOutMax=[]  ClampingZeroOutDataTypeStr=Inherit: Inherit via back propagation  ClampingZeroOutMin=[]  ClampingZeroOutMax=[]  FilterDenConstantOutDataTypeStr=Inherit: Inherit via back propagation  FilterDenConstantOutMin=[]  FilterDenConstantOutMax=[]  PCopyOutDataTypeStr=Inherit: Inherit via back propagation  PCopyOutMin=[]  PCopyOutMax=[]  NCopyOutDataTypeStr=Inherit: Inherit via back propagation  NCopyOutMin=[]  NCopyOutMax=[]  IntegratorContinuousStateAttributes=''  IntegratorStateMustResolveToSignalObject=off  IntegratorRTWStateStorageClass=Auto  FilterContinuousStateAttributes=''  FilterStateMustResolveToSignalObject=off  FilterRTWStateStorageClass=Auto  ParallelPVariant=InternalParameters  IdealPVariant=Disabled  IVariant=InternalParameters  DVariant=InternalParameters  IntegratorVariant=Discrete  SatVariant=Disabled  AWVariant=Passthrough  PCopyVariant=Disabled  TRVariant=Disabled  FdbkBlocksVariant=Forward  IdealPFdbkVariant=Disabled  SatFdbkVariant=Disabled  DerivativeFilterVariant=ForwardEulerFilter  NVariant=InternalParameters  NCopyVariant=Disabled  FilterICVariant=InternalICsFilter  IntegratorICVariant=InternalICs  ExternalResetVariant=Disabled  TRSumVariant=Passthrough  SumFdbkVariant=Disabled  SumVariant=Sum_PID  TsampFilterVariant=InternalTs  TsampNgainVariant=Passthrough  TsampIntegralVariant=Disabled_SignalSpec  ExternalSaturationOutDataTypeStr=Inherit: Same as second input
      settings: LibrarySourceBlock=simulink/Discrete/Discrete PID Controller
  cfblk5 : DiscreteStateSpace
  cfblk6 : simulink/Discrete/Difference  ICPrevInput=0.0  OutMin=[]  OutMax=[]  OutDataTypeStr=Inherit: Inherit via back propagation  OutDataType=fixdt(1, 16)  OutScaling=2^-10  DoSatur=off
  cfblk7 : Constant  Value=[-812243381.082024]  SampleTime=1
  cfblk8 : Constant  Value=[854735168.793008]  SampleTime=1
  cfblk2 : Outport
  cfblk11 : Outport  Port=2
  wires:
  cfblk3/1 -> cfblk4/1
  cfblk8/1 -> cfblk5/1
  cfblk10/1 -> cfblk6/1
  cfblk7/1 -> cfblk11/1
  cfblk9/1 -> cfblk2/1
  cfblk4/1 -> cfblk12/1
  cfblk12/1 -> cfblk3/1

== system model/cfblk69/cfblk8 ==
  cfblk1 : Inport
  cfblk8 : Inport  Port=2
  cfblk9 : Inport  Port=3
  cfblk10 : Inport  Port=4
  cfblk11 : Inport  Port=5
  cfblk3 : DiscreteIntegrator  ICPrevOutput=DiscIntNeverNeededParam  ICPrevScaledInput=DiscIntNeverNeededParam
  cfblk4 : Abs  SaturateOnIntegerOverflow=off
  cfblk5 : ComplexToRealImag
  cfblk6 : simulink/Math Operations/MinMax Running Resettable  Function=min  vinit=0.0
  cfblk7 : Sum  Inputs=+
  cfblk2 : Outport
  cfblk12 : Outport  Port=2
  wires:
  cfblk7/1 -> cfblk12/1
  cfblk11/1 -> cfblk5/1
  cfblk3/1 -> cfblk4/1
  cfblk9/1 -> cfblk6/1
  cfblk5/1 -> cfblk6/2
  cfblk4/1 -> cfblk7/1
  cfblk6/1 -> cfblk2/1
  cfblk5/2 -> cfblk3/1

== system model/cfblk69/cfblk9 ==
  cfblk1 : Inport
  cfblk12 : Inport  Port=2
  cfblk10 : Sqrt
  cfblk11 : Math  Operator=rem
  cfblk15 : Delay  SampleTime=1
  cfblk16 : Delay  SampleTime=1
  cfblk3 : DiscreteZeroPole  Poles=[0 0.5]  Gain=1
  cfblk4 : Delay  ShowEnablePort=on  SampleTime=1
      settings: InputPortMap=u0,e6
  cfblk5 : Sin  TimeSource=Use external signal  SampleTime=0
  cfblk6 : DotProduct  OutDataTypeStr=Inherit: Inherit via internal rule
  cfblk7 : Assignment  DiagnosticForDimensions=Warning  IndexOptions=Index vector (dialog)  Indices=1  OutputSizes=1
  cfblk8 : Sum  Inputs=|++
  cfblk9 : ComplexToRealImag
  cfblk2 : Outport
  cfblk13 : Outport  Port=2
  cfblk14 : Outport  Port=3
  wires:
  cfblk4/1 -> cfblk11/1, cfblk16/1
  cfblk1/1 -> cfblk7/1, cfblk8/2
  cfblk9/1 -> cfblk6/2
  cfblk7/1 -> cfblk5/1, cfblk4/2
  cfblk12/1 -> cfblk10/1
  cfblk9/2 -> cfblk14/1
  cfblk5/1 -> cfblk8/1
  cfblk10/1 -> cfblk2/1, cfblk13/1
  cfblk6/1 -> cfblk3/1
  cfblk3/1 -> cfblk4/1
  cfblk8/1 -> cfblk9/1, cfblk11/2
  cfblk11/1 -> cfblk15/1
  cfblk15/1 -> cfblk6/1
  cfblk16/1 -> cfblk7/2

== system model/cfblk70/cfblk10 ==
  cfblk1 : Inport
  cfblk10 : Delay  SampleTime=1
  cfblk3 : DiscreteZeroPole  Poles=[0 0.5]  Gain=1
  cfblk4 : Gain  Gain=[-404484764.544552]
  cfblk5 : Abs  SaturateOnIntegerOverflow=off
  cfblk6 : Trigonometry
  cfblk7 : Signum
  cfblk8 : Constant  Value=[-856759673.840609]  SampleTime=1
  cfblk9 : Constant  Value=[63198389.932601]  SampleTime=1
  cfblk2 : Outport
  wires:
  cfblk6/1 -> cfblk4/1
  cfblk3/1 -> cfblk7/1
  cfblk9/1 -> cfblk6/1
  cfblk5/1 -> cfblk2/1
  cfblk1/1 -> cfblk5/1
  cfblk7/1 -> cfblk10/1
  cfblk10/1 -> cfblk3/1

== system model/cfblk70/cfblk11 ==
  cfblk1 : Inport
  cfblk10 : Delay  SampleTime=1
  cfblk3 : DiscreteStateSpace
  cfblk4 : Product  Inputs=*
  cfblk5 : Polyval  Coefs=[ +2.081618890e-019, -1.441693666e-014, +4.719686976e-010, -8.536869453e-006, +1.621573104e-001, -8.087801117e+001 ]
  cfblk6 : Abs  SaturateOnIntegerOverflow=off
  cfblk7 : Trigonometry
  cfblk8 : simulink/Math Operations/Slider Gain  gain=1  low=0  high=2
  cfblk9 : Constant  Value=[326549079.533010]  SampleTime=1
  cfblk2 : Outport
  wires:
  cfblk1/1 -> cfblk4/1
  cfblk3/1 -> cfblk6/1
  cfblk4/1 -> cfblk8/1
  cfblk8/1 -> cfblk5/1
  cfblk9/1 -> cfblk7/1
  cfblk5/1 -> cfblk2/1
  cfblk6/1 -> cfblk10/1
  cfblk10/1 -> cfblk3/1

== system model/cfblk70/cfblk12 ==
  cfblk1 : Inport
  cfblk9 : Inport  Port=2
  cfblk12 : Delay  SampleTime=1
  cfblk3 : DiscreteStateSpace
  cfblk4 : Signum
  cfblk5 : PermuteDimensions
  cfblk6 : Signum
  cfblk7 : ComplexToMagnitudeAngle
  cfblk8 : Bias  Bias=[316908285.865711]  SaturateOnIntegerOverflow=off
  cfblk2 : Outport
  cfblk10 : Outport  Port=2
  cfblk11 : Outport  Port=3
  wires:
  cfblk6/1 -> cfblk10/1
  cfblk3/1 -> cfblk8/1
  cfblk9/1 -> cfblk5/1
  cfblk1/1 -> cfblk11/1
  cfblk5/1 -> cfblk6/1
  cfblk8/1 -> cfblk7/1
  cfblk7/1 -> cfblk2/1
  cfblk7/2 -> cfblk4/1
  cfblk4/1 -> cfblk12/1
  cfblk12/1 -> cfblk3/1

== system model/cfblk70/cfblk13 ==
  cfblk1 : Inport
  cfblk10 : Inport  Port=2
  cfblk11 : Inport  Port=3
  cfblk12 : Inport  Port=4
  cfblk14 : Delay  SampleTime=1
  cfblk3 : slpidlib/PID Controller  Controller=PID  Form=Parallel  TimeDomain=Discrete-time  UseExternalTs=off  SampleTime=1  IntegratorMethod=Forward Euler  FilterMethod=Forward Euler  ControllerParametersSource=internal  P=1  I=1  UseKiTs=off  D=0  N=100  UseFilter=on  TunerSelectOption=Transfer Function Based (PID Tuner App)  InitialConditionSource=internal  InitialConditionForIntegrator=0  InitialConditionForFilter=0  DifferentiatorICPrevScaledInput=0  ExternalReset=none  TrackingMode=off  Kt=1  LimitOutput=off  SatLimitsSource=internal  UpperSaturationLimit=inf  LowerSaturationLimit=-inf  LinearizeAsGain=off  AntiWindupMode=none  Kb=1  LimitIntegrator=off  UpperIntegratorSaturationLimit=inf  LowerIntegratorSaturationLimit=-inf  POutMin=[]  POutMax=[]  IOutMin=[]  IOutMax=[]  DOutMin=[]  DOutMax=[]  NOutMin=[]  NOutMax=[]  SumOutMin=[]  SumOutMax=[]  SaturationOutMin=[]  SaturationOutMax=[]  PParamMin=[]  PParamMax=[]  IParamMin=[]  IParamMax=[]  DParamMin=[]  DParamMax=[]  NParamMin=[]  NParamMax=[]  KbParamMin=[]  KbParamMax=[]  KtParamMin=[]  KtParamMax=[]  KbOutMin=[]  KbOutMax=[]  KtOutMin=[]  KtOutMax=[]  IntegratorOutMin=[]  IntegratorOutMax=[]  FilterOutMin=[]  FilterOutMax=[]  SumI1OutMin=[]  SumI1OutMax=[]  SumI2OutMin=[]  SumI2OutMax=[]  SumI3OutMin=[]  SumI3OutMax=[]  SumI4OutMin=[]  SumI4OutMax=[]  SumDOutMin=[]  SumDOutMax=[]  DifferentiatorOutMin=[]  DifferentiatorOutMax=[]  FilterDiffOutCoefMin=[]  FilterDiffOutCoefMax=[]  ReciprocalOutMin=[]  ReciprocalOutMax=[]  SumDenOutMin=[]  SumDenOutMax=[]  SumNumOutMin=[]  SumNumOutMax=[]  DivideOutMin=[]  DivideOutMax=[]  UdiffTsProdOutMin=[]  UdiffTsProdOutMax=[]  NTsProdOutMin=[]  NTsProdOutMax=[]  UintegralTsProdOutMin=[]  UintegralTsProdOutMax=[]  UngainTsProdOutMin=[]  UngainTsProdOutMax=[]  ClampingZeroOutDataTypeStr=Inherit: Inherit via back propagation  ClampingZeroOutMin=[]  ClampingZeroOutMax=[]  FilterDenConstantOutDataTypeStr=Inherit: Inherit via back propagation  FilterDenConstantOutMin=[]  FilterDenConstantOutMax=[]  PCopyOutDataTypeStr=Inherit: Inherit via back propagation  PCopyOutMin=[]  PCopyOutMax=[]  NCopyOutDataTypeStr=Inherit: Inherit via back propagation  NCopyOutMin=[]  NCopyOutMax=[]  IntegratorContinuousStateAttributes=''  IntegratorStateMustResolveToSignalObject=off  IntegratorRTWStateStorageClass=Auto  FilterContinuousStateAttributes=''  FilterStateMustResolveToSignalObject=off  FilterRTWStateStorageClass=Auto  ParallelPVariant=InternalParameters  IdealPVariant=Disabled  IVariant=InternalParameters  DVariant=InternalParameters  IntegratorVariant=Discrete  SatVariant=Disabled  AWVariant=Passthrough  PCopyVariant=Disabled  TRVariant=Disabled  FdbkBlocksVariant=Forward  IdealPFdbkVariant=Disabled  SatFdbkVariant=Disabled  DerivativeFilterVariant=ForwardEulerFilter  NVariant=InternalParameters  NCopyVariant=Disabled  FilterICVariant=InternalICsFilter  IntegratorICVariant=InternalICs  ExternalResetVariant=Disabled  TRSumVariant=Passthrough  SumFdbkVariant=Disabled  SumVariant=Sum_PID  TsampFilterVariant=InternalTs  TsampNgainVariant=Passthrough  TsampIntegralVariant=Disabled_SignalSpec  ExternalSaturationOutDataTypeStr=Inherit: Same as second input
      settings: LibrarySourceBlock=simulink/Discrete/Discrete PID Controller
  cfblk4 : PropagationDelay  SampleTime=1
  cfblk5 : Delay  ShowEnablePort=on  SampleTime=1
      settings: InputPortMap=u0,e6
  cfblk6 : UnitDelay  HasFrameUpgradeWarning=on
  cfblk7 : MinMax  Inputs=2
  cfblk8 : ComplexToMagnitudeAngle
  cfblk9 : Constant  Value=[59318251.157664]  SampleTime=1
  cfblk2 : Outport
  cfblk13 : Outport  Port=2
  wires:
  cfblk12/1 -> cfblk7/1
  cfblk11/1 -> cfblk5/1
  cfblk10/1 -> cfblk4/2
  cfblk3/1 -> cfblk7/2
  cfblk1/1 -> cfblk3/1
  cfblk5/1 -> cfblk2/1
  cfblk9/1 -> cfblk5/2
  cfblk4/1 -> cfblk8/1
  cfblk7/1 -> cfblk13/1
  cfblk8/1 -> cfblk6/1
  cfblk6/1 -> cfblk14/1
  cfblk14/1 -> cfblk4/1

== system model/cfblk70/cfblk14 ==
  cfblk1 : Inport
  cfblk12 : Inport  Port=2
  cfblk13 : Inport  Port=3
  cfblk10 : Sqrt
  cfblk11 : Constant  Value=[160043659.324022]  SampleTime=1
  cfblk16 : Delay  SampleTime=1
  cfblk3 : simulink/Discrete/Difference  ICPrevInput=0.0  OutMin=[]  OutMax=[]  OutDataTypeStr=Inherit: Inherit via back propagation  OutDataType=fixdt(1, 16)  OutScaling=2^-10  DoSatur=off
  cfblk4 : Sin  TimeSource=Use external signal  SampleTime=0
  cfblk5 : Abs  SaturateOnIntegerOverflow=off
  cfblk6 : Math  Operator=square
  cfblk7 : simulink/Math Operations/MinMax Running Resettable  Function=min  vinit=0.0
  cfblk8 : ComplexToRealImag
  cfblk9 : PermuteDimensions
  cfblk2 : Outport
  cfblk14 : Outport  Port=2
  cfblk15 : Outport  Port=3
  wires:
  cfblk11/1 -> cfblk2/1
  cfblk10/1 -> cfblk9/1
  cfblk8/1 -> cfblk10/1
  cfblk3/1 -> cfblk14/1
  cfblk12/1 -> cfblk7/1
  cfblk13/1 -> cfblk5/1
  cfblk1/1 -> cfblk7/2
  cfblk6/1 -> cfblk8/1
  cfblk4/1 -> cfblk15/1
  cfblk5/1 -> cfblk4/1
  cfblk7/1 -> cfblk3/1
  cfblk9/1 -> cfblk16/1
  cfblk16/1 -> cfblk6/1

== system model/cfblk70/cfblk9 ==
  cfblk1 : Inport
  cfblk10 : Inport  Port=2
  cfblk11 : Inport  Port=3
  cfblk3 : Abs  SaturateOnIntegerOverflow=off
  cfblk4 : Sum  Inputs=|++
  cfblk5 : ComplexToRealImag
  cfblk6 : Product  Inputs=**
  cfblk7 : Bias  Bias=[-665396221.822448]  SaturateOnIntegerOverflow=off
  cfblk8 : Constant  Value=[380681705.872159]  SampleTime=1
  cfblk9 : Constant  Value=[228527759.416245]  SampleTime=1
  cfblk2 : Outport
  wires:
  cfblk6/1 -> cfblk2/1
  cfblk5/1 -> cfblk7/1
  cfblk9/1 -> cfblk3/1
  cfblk3/1 -> cfblk4/1
  cfblk7/1 -> cfblk4/2
  cfblk8/1 -> cfblk6/1
  cfblk10/1 -> cfblk6/2
  cfblk1/1 -> cfblk5/1
